simulink model "Malabanan_Problem8"  (R2023b)
settings: Solver=VariableStepAuto  StartTime=0.0  StopTime=20  RelTol=1e-3
values from neighbouring files (symbols this model uses):
  G_den8 = [1 3 5 7 9 1]    [MALABANAN_NO8.m]
  G_num8 = [10 8 6 4 2]    [MALABANAN_NO8.m]
settings Model: Creator=Asus  LastModifiedBy=USER

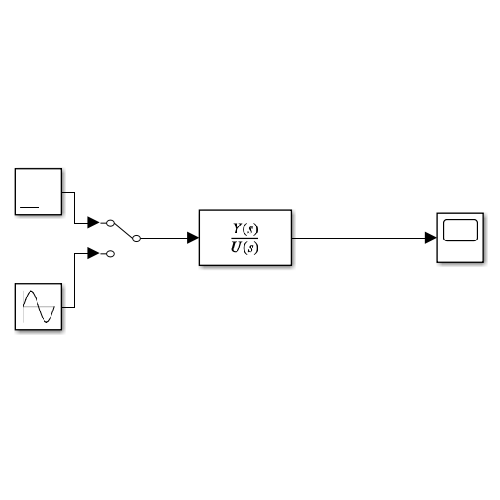
[thumbnail: Simulink's stored preview of the top-level diagram]
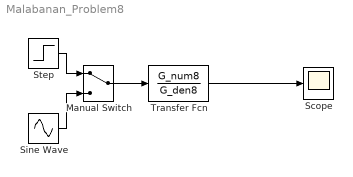
== system Malabanan_Problem8 ==
  Manual Switch : ManualSwitch
  Scope : Scope
  Sine Wave : Sin  SampleTime=0
  Step : Step  Time=0  SampleTime=0
  Transfer Fcn : TransferFcn  Numerator=G_num8  Denominator=G_den8
  wires:
  Step/1 -> Manual Switch/1
  Sine Wave/1 -> Manual Switch/2
  Manual Switch/1 -> Transfer Fcn/1
  Transfer Fcn/1 -> Scope/1
